simulink model "ros2webots_localization_model_cg"  (R2023a)
settings: Solver=FixedStepDiscrete  StartTime=0.0  StopTime=inf  FixedStep=0.05  RelTol=1e-3  EnableMultiTasking=on
model workspace (MAT data in the model file):
  Logfile_Data_Object = robotics.ros.BagSelection
  Logfile_Data_Object.FilePath = '\\wsl.localhost\ubuntu\home\mjavadzallaghi\ros2_ws\ros2webots\baglog\rosbot_data_20240125_225927.bag'
  Logfile_Data_Object.StartTime = 1706210981.23
  Logfile_Data_Object.EndTime = 1706211126.25
  Logfile_Data_Object.NumMessages = 508
  Logfile_Data_Object.AvailableTopics = table
  Logfile_Data_Object.AvailableTopics.data{1} = [73; 435]
  Logfile_Data_Object.AvailableTopics.data{2} = categorical
  Logfile_Data_Object.AvailableTopics.data{2}.categoryNames = {'geometry_msgs/Twist'; 'sensor_msgs/Imu'}
  Logfile_Data_Object.AvailableTopics.data{2}.codes = [1; 2]
  Logfile_Data_Object.AvailableTopics.data{3}{1} = 'geometry_msgs/Vector3 Linear
    |   double X
    |   double Y
    |   double Z
    | geometry_msgs/Vector3 Angular
    |   double X
    |   double Y
    |   double Z
    | '
  Logfile_Data_Object.AvailableTopics.data{3}{2} = 'std_msgs/Header Header
    |   uint32 Seq
    |   Time Stamp
    |   char FrameId
    | geometry_msgs/Quaternion Orientation
    |   double X
    |   double Y
    |   double Z
    |   double W
    | double[9] OrientationCovariance
    | geometry_msgs/Vector3 AngularVelocity
    |   double X
    |   double Y
    |   double Z
    | double[9] AngularVelocityCovariance
    | geometry_msgs/Vector3 LinearAcceleration
    |   double X
    |   double Y
    |   double Z
    | double[9] LinearAccelerationCovariance
    | '
  Logfile_Data_Object.AvailableTopics.ndims = 2
  Logfile_Data_Object.AvailableTopics.nrows = 2
  Logfile_Data_Object.AvailableTopics.rownames = {'/webots/rosbot/command_vel'; '/webots/rosbot/imu'}
  Logfile_Data_Object.AvailableTopics.nvars = 3
  Logfile_Data_Object.AvailableTopics.varnames = {'NumMessages', 'MessageType', 'MessageDefinition'}
  Logfile_Data_Object.AvailableTopics.props.useVariableNamesOriginal = 0
  Logfile_Data_Object.AvailableTopics.props.useDimensionNamesOriginal = 0
  Logfile_Data_Object.AvailableTopics.props.CustomProps = struct()
  Logfile_Data_Object.AvailableTopics.props.VariableCustomProps = struct()
  Logfile_Data_Object.AvailableTopics.props.versionSavedFrom = 4
  Logfile_Data_Object.AvailableTopics.props.minCompatibleVersion = 1
  Logfile_Data_Object.AvailableTopics.props.incompatibilityMsg = ''
  Logfile_Data_Object.AvailableTopics.props.VersionSavedFrom = 4
  Logfile_Data_Object.AvailableTopics.props.Description = ''
  Logfile_Data_Object.AvailableTopics.props.VariableNamesOriginal = {}
  Logfile_Data_Object.AvailableTopics.props.DimensionNames = {'Row', 'Variables'}
  Logfile_Data_Object.AvailableTopics.props.DimensionNamesOriginal = {}
  Logfile_Data_Object.AvailableTopics.props.UserData = []
  Logfile_Data_Object.AvailableTopics.props.VariableDescriptions = {}
  Logfile_Data_Object.AvailableTopics.props.VariableUnits = {}
  Logfile_Data_Object.AvailableTopics.props.VariableContinuity = {}
  Logfile_Data_Object.MessageList = table
  Logfile_Data_Object.MessageList.data{1} = [1706210981.23 1706210981.23 1706210981.23 1706210983.05 1706210983.38 1706210983.7 1706210984.04 1706210984.38 1706210984.72 1706210985.07 1706210985.41 1706210985.73 ... (508 elements, 508x1)]
  Logfile_Data_Object.MessageList.data{2} = categorical
  Logfile_Data_Object.MessageList.data{2}.categoryNames = {'/webots/rosbot/command_vel'; '/webots/rosbot/imu'}
  Logfile_Data_Object.MessageList.data{2}.codes = [1; 1; 1; 2; 2; 2; 2; 2; 2; 2; 2; 1; 1; 1; 2; 2; 2; 2; 2; 2; 2; 2; 2; 2; 2; 2; 2; 2; 2; 2; 2; 2; 2; 2; 2; 2; 2; 2; 1; 1; 1; 2; 2; 2; 2; 2; 2; 2; 2; 2; 2; 2; 2; 2; 2; 2; 2; 2; 2; 2; 2; 2; 2; 2; 2; 2; 2; 1; 1; 1; 2; 2; 2; 2; 2; 2; 2; 2; 2; 2; 2; 2; 2; 2; 2; 2; 2; 2; 2; 2; 2; 1; 1; 1; 2; 2; 2; 2; 2; 2; 2; 2; 2; 2; 2; 2; 2; 2; 2; 2; 2; 2; 2; 2; 2; 2; 2; 2; 1; 1; 2; 1; 2; 2; 2; 2; 2; 2; 2; 2; 2; 2; 2; 2; 2; 2; 2; 2; 2; 2; 2; 2; 2; 2; 2; 2; 2; 2; 2; 2; 2; 2; 2; 2; 2; 2; 2; 2; 2; 2; 2; 2; 2; 2; 2; 2; 1; 1; 1; 2; 2; 2; 2; 2; 2; 2; 2; 2; 2; 2; 2; 2; 2; 2; 2; 2; 2; 2; 2; 2; 2; 2; 2; 1; 1; 1; 2; 2; 2; 2; 2; 2; 2; 2; 2; 2; 2; 2; 2; 2; 2; 2; 2; 2; 2; 2; 2; 2; 2; 2; 2; 2; 2; 1; 1; 1; 2; 2; 2; 2; 2; 2; 2; 2; 2; 2; 2; 2; 2; 2; 2; 2; 2; 2; 2; 2; 2; 2; 2; 2; 2; 2; 1; 1; 1; 2; 2; 2; 2; 2; 2; 2; 2; 2; 2; 2; 2; 2; 2; 2; 2; 2; 2; 2; 2; 1; 1; 1; 2; 2; 2; 2; 2; 2; 2; 2; 2; 2; 2; 2; 2; 2; 2; 2; 2; 2; 2; 2; 2; 2; 2; 2; 2; 1; 1; 1; 2; 2; 2; 2; 2; 2; 2; 1; 1; 2; 1; 2; 2; 2; 2; 2; 2; 1; 1; 1; 2; 2; 2; 2; 2; 2; 2; 2; 2; 2; 2; 2; 1; 1; 1; 2; 2; 2; 2; 2; 2; 2; 2; 2; 2; 2; 2; 2; 2; 2; 2; 2; 2; 2; 1; 1; 1; 2; 2; 2; 2; 2; 2; 2; 2; 2; 1; 1; 1; 2; 2; 2; 2; 2; 2; 2; 2; 2; 2; 2; 2; 1; 1; 1; 2; 2; 2; 2; 2; 2; 1; 1; 1; 2; 2; 2; 2; 2; 2; 2; 2; 2; 2; 2; 2; 1; 1; 1; 2; 2; 2; 2; 2; 2; 2; 2; 2; 2; 1; 1; 1; 2; 2; 2; 2; 2; 2; 2; 2; 2; 2; 1; 1; 1; 2; 2; 2; 2; 2; 2; 2; 1; 1; 1; 2; 2; 2; 2; 2; 2; 2; 2; 2; 2; 2; 2; 2; 2; 2; 2; 1; 1; 1; 2; 2; 2; 2; 2; 2; 2; 2; 2; 2; 2; 2; 2; 2; 2; 2; 1; 2; 2; 2; 2; 2; 2; 2; 2; 2; 2; 2; 2; 2; 2; 2; 2; 2; 2; 2; 2; 2; 2]
  Logfile_Data_Object.MessageList.data{3} = categorical
  Logfile_Data_Object.MessageList.data{3}.categoryNames = {'geometry_msgs/Twist'; 'sensor_msgs/Imu'}
  Logfile_Data_Object.MessageList.data{3}.codes = [1; 1; 1; 2; 2; 2; 2; 2; 2; 2; 2; 1; 1; 1; 2; 2; 2; 2; 2; 2; 2; 2; 2; 2; 2; 2; 2; 2; 2; 2; 2; 2; 2; 2; 2; 2; 2; 2; 1; 1; 1; 2; 2; 2; 2; 2; 2; 2; 2; 2; 2; 2; 2; 2; 2; 2; 2; 2; 2; 2; 2; 2; 2; 2; 2; 2; 2; 1; 1; 1; 2; 2; 2; 2; 2; 2; 2; 2; 2; 2; 2; 2; 2; 2; 2; 2; 2; 2; 2; 2; 2; 1; 1; 1; 2; 2; 2; 2; 2; 2; 2; 2; 2; 2; 2; 2; 2; 2; 2; 2; 2; 2; 2; 2; 2; 2; 2; 2; 1; 1; 2; 1; 2; 2; 2; 2; 2; 2; 2; 2; 2; 2; 2; 2; 2; 2; 2; 2; 2; 2; 2; 2; 2; 2; 2; 2; 2; 2; 2; 2; 2; 2; 2; 2; 2; 2; 2; 2; 2; 2; 2; 2; 2; 2; 2; 2; 1; 1; 1; 2; 2; 2; 2; 2; 2; 2; 2; 2; 2; 2; 2; 2; 2; 2; 2; 2; 2; 2; 2; 2; 2; 2; 2; 1; 1; 1; 2; 2; 2; 2; 2; 2; 2; 2; 2; 2; 2; 2; 2; 2; 2; 2; 2; 2; 2; 2; 2; 2; 2; 2; 2; 2; 2; 1; 1; 1; 2; 2; 2; 2; 2; 2; 2; 2; 2; 2; 2; 2; 2; 2; 2; 2; 2; 2; 2; 2; 2; 2; 2; 2; 2; 2; 1; 1; 1; 2; 2; 2; 2; 2; 2; 2; 2; 2; 2; 2; 2; 2; 2; 2; 2; 2; 2; 2; 2; 1; 1; 1; 2; 2; 2; 2; 2; 2; 2; 2; 2; 2; 2; 2; 2; 2; 2; 2; 2; 2; 2; 2; 2; 2; 2; 2; 2; 1; 1; 1; 2; 2; 2; 2; 2; 2; 2; 1; 1; 2; 1; 2; 2; 2; 2; 2; 2; 1; 1; 1; 2; 2; 2; 2; 2; 2; 2; 2; 2; 2; 2; 2; 1; 1; 1; 2; 2; 2; 2; 2; 2; 2; 2; 2; 2; 2; 2; 2; 2; 2; 2; 2; 2; 2; 1; 1; 1; 2; 2; 2; 2; 2; 2; 2; 2; 2; 1; 1; 1; 2; 2; 2; 2; 2; 2; 2; 2; 2; 2; 2; 2; 1; 1; 1; 2; 2; 2; 2; 2; 2; 1; 1; 1; 2; 2; 2; 2; 2; 2; 2; 2; 2; 2; 2; 2; 1; 1; 1; 2; 2; 2; 2; 2; 2; 2; 2; 2; 2; 1; 1; 1; 2; 2; 2; 2; 2; 2; 2; 2; 2; 2; 1; 1; 1; 2; 2; 2; 2; 2; 2; 2; 1; 1; 1; 2; 2; 2; 2; 2; 2; 2; 2; 2; 2; 2; 2; 2; 2; 2; 2; 1; 1; 1; 2; 2; 2; 2; 2; 2; 2; 2; 2; 2; 2; 2; 2; 2; 2; 2; 1; 2; 2; 2; 2; 2; 2; 2; 2; 2; 2; 2; 2; 2; 2; 2; 2; 2; 2; 2; 2; 2; 2]
  Logfile_Data_Object.MessageList.data{4} = [5438 5532 5626 5720 6078 6436 6794 7152 7510 7868 8226 8584 ... (508 elements, 508x1)]
  Logfile_Data_Object.MessageList.ndims = 2
  Logfile_Data_Object.MessageList.nrows = 508
  Logfile_Data_Object.MessageList.nvars = 4
  Logfile_Data_Object.MessageList.varnames = {'Time', 'Topic', 'MessageType', 'FileOffset'}
  Logfile_Data_Object.MessageList.props.useVariableNamesOriginal = 0
  Logfile_Data_Object.MessageList.props.useDimensionNamesOriginal = 0
  Logfile_Data_Object.MessageList.props.CustomProps = struct()
  Logfile_Data_Object.MessageList.props.VariableCustomProps = struct()
  Logfile_Data_Object.MessageList.props.versionSavedFrom = 4
  Logfile_Data_Object.MessageList.props.minCompatibleVersion = 1
  Logfile_Data_Object.MessageList.props.incompatibilityMsg = ''
  Logfile_Data_Object.MessageList.props.VersionSavedFrom = 4
  Logfile_Data_Object.MessageList.props.Description = ''
  Logfile_Data_Object.MessageList.props.VariableNamesOriginal = {}
  Logfile_Data_Object.MessageList.props.DimensionNames = {'Row', 'Variables'}
  Logfile_Data_Object.MessageList.props.DimensionNamesOriginal = {}
  Logfile_Data_Object.MessageList.props.UserData = []
  Logfile_Data_Object.MessageList.props.VariableDescriptions = {}
  Logfile_Data_Object.MessageList.props.VariableUnits = {}
  Logfile_Data_Object.MessageList.props.VariableContinuity = {}
  Logfile_Data_Object.RawMessageBuffer = containers.Map
  Logfile_Data_Object.RawMessageBuffer.serialization.keys = {}
  Logfile_Data_Object.RawMessageBuffer.serialization.values = {}
  Logfile_Data_Object.RawMessageBuffer.serialization.uniformity = 0
  Logfile_Data_Object.RawMessageBuffer.serialization.keyType = 'char'
  Logfile_Data_Object.RawMessageBuffer.serialization.valueType = 'any'
  Logfile_Data_Object.ImgMessageBuffer = containers.Map
  Logfile_Data_Object.ImgMessageBuffer.serialization.keys = {}
  Logfile_Data_Object.ImgMessageBuffer.serialization.values = {}
  Logfile_Data_Object.ImgMessageBuffer.serialization.uniformity = 0
  Logfile_Data_Object.ImgMessageBuffer.serialization.keyType = 'char'
  Logfile_Data_Object.ImgMessageBuffer.serialization.valueType = 'any'
  Logfile_Data_Object.PointCloudBuffer = containers.Map
  Logfile_Data_Object.PointCloudBuffer.serialization.keys = {}
  Logfile_Data_Object.PointCloudBuffer.serialization.values = {}
  Logfile_Data_Object.PointCloudBuffer.serialization.uniformity = 0
  Logfile_Data_Object.PointCloudBuffer.serialization.keyType = 'char'
  Logfile_Data_Object.PointCloudBuffer.serialization.valueType = 'any'
  Logfile_Data_Object.LaserScanBuffer = containers.Map
  Logfile_Data_Object.LaserScanBuffer.serialization.keys = {}
  Logfile_Data_Object.LaserScanBuffer.serialization.values = {}
  Logfile_Data_Object.LaserScanBuffer.serialization.uniformity = 0
  Logfile_Data_Object.LaserScanBuffer.serialization.keyType = 'char'
  Logfile_Data_Object.LaserScanBuffer.serialization.valueType = 'any'
  Logfile_Data_Object.TopicTypeMap = containers.Map
  Logfile_Data_Object.TopicTypeMap.serialization.keys = {'/webots/rosbot/command_vel', '/webots/rosbot/imu'}
  Logfile_Data_Object.TopicTypeMap.serialization.values = {'geometry_msgs/Twist', 'sensor_msgs/Imu'}
  Logfile_Data_Object.TopicTypeMap.serialization.uniformity = 1
  Logfile_Data_Object.TopicTypeMap.serialization.keyType = 'char'
  Logfile_Data_Object.TopicTypeMap.serialization.valueType = 'char'
  Logfile_Data_Object.TopicDefinitionMap = containers.Map
  Logfile_Data_Object.TopicDefinitionMap.serialization.keys = {'/webots/rosbot/command_vel', '/webots/rosbot/imu'}
  Logfile_Data_Object.TopicDefinitionMap.serialization.values{1} = 'geometry_msgs/Vector3 Linear
    |   double X
    |   double Y
    |   double Z
    | geometry_msgs/Vector3 Angular
    |   double X
    |   double Y
    |   double Z
    | '
  Logfile_Data_Object.TopicDefinitionMap.serialization.values{2} = 'std_msgs/Header Header
    |   uint32 Seq
    |   Time Stamp
    |   char FrameId
    | geometry_msgs/Quaternion Orientation
    |   double X
    |   double Y
    |   double Z
    |   double W
    | double[9] OrientationCovariance
    | geometry_msgs/Vector3 AngularVelocity
    |   double X
    |   double Y
    |   double Z
    | double[9] AngularVelocityCovariance
    | geometry_msgs/Vector3 LinearAcceleration
    |   double X
    |   double Y
    |   double Z
    | double[9] LinearAccelerationCovariance
    | '
  Logfile_Data_Object.TopicDefinitionMap.serialization.uniformity = 1
  Logfile_Data_Object.TopicDefinitionMap.serialization.keyType = 'char'
  Logfile_Data_Object.TopicDefinitionMap.serialization.valueType = 'char'
  Logfile_Data_Object.messageTypeMap = containers.Map
  Logfile_Data_Object.messageTypeMap.serialization.keys = {}
  Logfile_Data_Object.messageTypeMap.serialization.values = {}
  Logfile_Data_Object.messageTypeMap.serialization.uniformity = 0
  Logfile_Data_Object.messageTypeMap.serialization.keyType = 'char'
  Logfile_Data_Object.messageTypeMap.serialization.valueType = 'any'
  Logfile_Data_Object.Parser = robotics.ros.internal.tf.TransformationTreeParser
  Logfile_Data_Object.Parser.UseObjectMsg = 1
  Logfile_Path = '\\wsl.localhost\ubuntu\home\mjavadzallaghi\ros2_ws\ros2webots\baglog\rosbot_data_20240125_225927.bag'
  Logfile_Playback_Duration = nan
  Logfile_Playback_Offset = nan
values from neighbouring files (symbols this model uses):
  wheel_based_localization_x_initial_coord = 0.0    [ros2webots_localization_model.sldd]
  wheel_based_localization_y_initial_coord = 0.0    [ros2webots_localization_model.sldd]
libraries: sharedtransform x1
settings Model: DataDictionary=ros2webots_localization_model.sldd  Creator=MJava  LastModifiedBy=MJava
settings SolverCC: AllowMultiTaskInputOutput=on  AutoInsertRateTranBlk=on
settings OptimizationCC: DefaultParameterBehavior=Inlined  EnhancedBackFolding=on  PassReuseOutputArgsAs=Individual arguments  ZeroExternalMemoryAtStartup=off  ZeroInternalMemoryAtStartup=off  MaxStackSize=64  OptimizeBlockOrder=speed  DifferentSizesBufferReuse=on  OptimizationCustomize=off  EfficientTunableParamExpr=on
settings DebuggingCC: ParameterTunabilityLossMsg=error
settings SFSimCC: MATLABDynamicMemAlloc=off  SimTargetLang=C++
settings RTWCC: Description=Embedded Coder  SystemTargetFile=ert.tlc  TemplateMakefile=ert_default_tmf  GenerateReport=on  Toolchain=Microsoft Visual C++ 2019 v16.0 | nmake (64-bit Windows)  BuildConfiguration=Faster Runs  LaunchReport=on  TargetLang=C++  GenerateWebview=on  GenerateCodeMetricsReport=on  CheckMdlBeforeBuild=Warning
settings CodeAppCC: ForceParamTrailComments=on  IgnoreCustomStorageClasses=off  OperatorAnnotations=on  SimulinkDataObjDesc=on  SFDataObjDesc=on  InsertBlockDesc=on
settings ERTTargetCC: TargetLangStandard=C++11 (ISO)  CodeInterfacePackaging=C++ class  RootIOFormat=Structure reference  ERTCustomFileTemplate=example_file_process.tlc

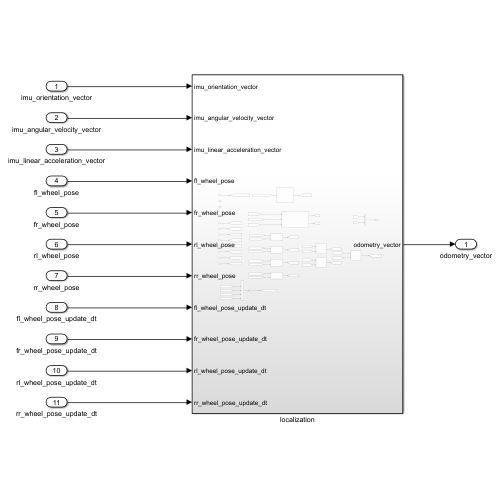
[thumbnail: Simulink's stored preview of the top-level diagram]
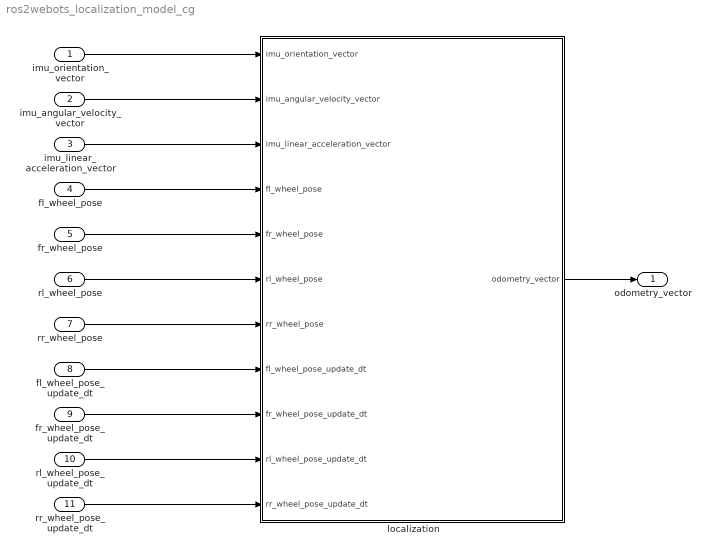
== system ros2webots_localization_model_cg ==
  imu_orientation_vector : Inport  OutDataTypeStr=double  PortDimensions=4
  imu_angular_velocity_vector : Inport  Port=2  OutDataTypeStr=double  PortDimensions=3
  imu_linear_acceleration_vector : Inport  Port=3  OutDataTypeStr=double  PortDimensions=3
  fl_wheel_pose : Inport  Port=4  OutDataTypeStr=double  PortDimensions=1
  fr_wheel_pose : Inport  Port=5  OutDataTypeStr=double  PortDimensions=1
  rl_wheel_pose : Inport  Port=6  OutDataTypeStr=double  PortDimensions=1
  rr_wheel_pose : Inport  Port=7  OutDataTypeStr=double  PortDimensions=1
  fl_wheel_pose_update_dt : Inport  Port=8  OutDataTypeStr=double  PortDimensions=1
  fr_wheel_pose_update_dt : Inport  Port=9  OutDataTypeStr=double  PortDimensions=1
  rl_wheel_pose_update_dt : Inport  Port=10  OutDataTypeStr=double  PortDimensions=1
  rr_wheel_pose_update_dt : Inport  Port=11  OutDataTypeStr=double  PortDimensions=1
  localization : Subsystem
  odometry_vector : Outport  OutDataTypeStr=double  PortDimensions=2
  wires:
  imu_orientation_vector/1 -> localization/1(imu_orientation_vector)
  imu_linear_acceleration_vector/1 -> localization/3(imu_linear_acceleration_vector)
  imu_angular_velocity_vector/1 -> localization/2(imu_angular_velocity_vector)
  rl_wheel_pose/1 -> localization/6(rl_wheel_pose)
  rr_wheel_pose/1 -> localization/7(rr_wheel_pose)
  fl_wheel_pose/1 -> localization/4(fl_wheel_pose)
  fr_wheel_pose/1 -> localization/5(fr_wheel_pose)
  rl_wheel_pose_update_dt/1 -> localization/10(rl_wheel_pose_update_dt)
  fr_wheel_pose_update_dt/1 -> localization/9(fr_wheel_pose_update_dt)
  fl_wheel_pose_update_dt/1 -> localization/8(fl_wheel_pose_update_dt)
  rr_wheel_pose_update_dt/1 -> localization/11(rr_wheel_pose_update_dt)
  localization/1(odometry_vector) -> odometry_vector/1

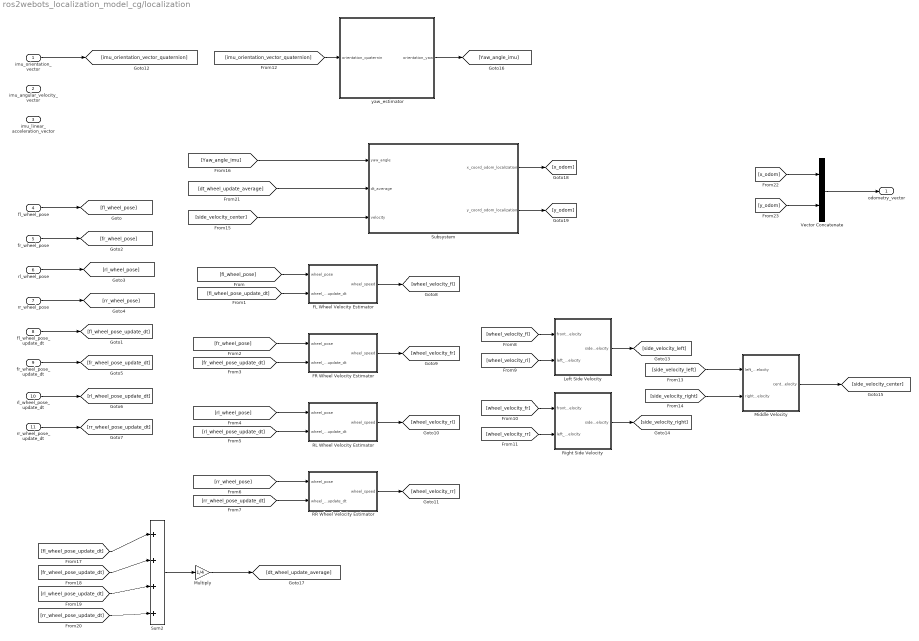
== system ros2webots_localization_model_cg/localization ==
  imu_orientation_vector : Inport  OutDataTypeStr=double  PortDimensions=4
  imu_angular_velocity_vector : Inport  Port=2  OutDataTypeStr=double  PortDimensions=3
  imu_linear_acceleration_vector : Inport  Port=3  OutDataTypeStr=double  PortDimensions=3
  fl_wheel_pose : Inport  Port=4
  fr_wheel_pose : Inport  Port=5
  rl_wheel_pose : Inport  Port=6
  rr_wheel_pose : Inport  Port=7
  fl_wheel_pose_update_dt : Inport  Port=8
  fr_wheel_pose_update_dt : Inport  Port=9
  rl_wheel_pose_update_dt : Inport  Port=10
  rr_wheel_pose_update_dt : Inport  Port=11
  FL Wheel Velocity Estimator : Subsystem
  FR Wheel Velocity Estimator : Subsystem
  Left Side Velocity : Subsystem
  Middle Velocity : Subsystem
  Multiply : Gain  Gain=1/4
  RL Wheel Velocity Estimator : Subsystem
  RR Wheel Velocity Estimator : Subsystem
  Right Side Velocity : Subsystem
  Subsystem : Subsystem
  Sum2 : Sum  Inputs=|++++
  Vector Concatenate : Concatenate
  yaw_estimator : Subsystem
  odometry_vector : Outport  PortDimensions=2
  wires:
  fl_wheel_pose_update_dt/1 -> [fl_wheel_pose_update_dt]
  [fl_wheel_pose] -> FL Wheel Velocity Estimator/1(wheel_pose)
  [fl_wheel_pose_update_dt] -> FL Wheel Velocity Estimator/2(wheel_pose_update_dt)
  fl_wheel_pose/1 -> [fl_wheel_pose]
  fr_wheel_pose/1 -> [fr_wheel_pose]
  rl_wheel_pose/1 -> [rl_wheel_pose]
  rr_wheel_pose/1 -> [rr_wheel_pose]
  fr_wheel_pose_update_dt/1 -> [fr_wheel_pose_update_dt]
  rl_wheel_pose_update_dt/1 -> [rl_wheel_pose_update_dt]
  rr_wheel_pose_update_dt/1 -> [rr_wheel_pose_update_dt]
  [fr_wheel_pose] -> FR Wheel Velocity Estimator/1(wheel_pose)
  [fr_wheel_pose_update_dt] -> FR Wheel Velocity Estimator/2(wheel_pose_update_dt)
  [rl_wheel_pose] -> RL Wheel Velocity Estimator/1(wheel_pose)
  [rl_wheel_pose_update_dt] -> RL Wheel Velocity Estimator/2(wheel_pose_update_dt)
  [rr_wheel_pose] -> RR Wheel Velocity Estimator/1(wheel_pose)
  [rr_wheel_pose_update_dt] -> RR Wheel Velocity Estimator/2(wheel_pose_update_dt)
  FL Wheel Velocity Estimator/1(wheel_speed) -> [wheel_velocity_fl]
  FR Wheel Velocity Estimator/1(wheel_speed) -> [wheel_velocity_fr]
  RL Wheel Velocity Estimator/1(wheel_speed) -> [wheel_velocity_rl]
  RR Wheel Velocity Estimator/1(wheel_speed) -> [wheel_velocity_rr]
  [wheel_velocity_fl] -> Left Side Velocity/1(front_wheel_velocity)
  [wheel_velocity_rl] -> Left Side Velocity/2(left_wheel_velocity)
  [wheel_velocity_fr] -> Right Side Velocity/1(front_wheel_velocity)
  [wheel_velocity_rr] -> Right Side Velocity/2(left_wheel_velocity)
  imu_orientation_vector/1 -> [imu_orientation_vector_quaternion]
  [imu_orientation_vector_quaternion] -> yaw_estimator/1(orientation_quaternin)
  Left Side Velocity/1(side_velocity) -> [side_velocity_left]
  Right Side Velocity/1(side_velocity) -> [side_velocity_right]
  [side_velocity_left] -> Middle Velocity/1(left_side_velocity)
  [side_velocity_right] -> Middle Velocity/2(right_side_velocity)
  Middle Velocity/1(center_velocity) -> [side_velocity_center]
  yaw_estimator/1(orientation_yaw) -> [Yaw_angle_imu]
  [fl_wheel_pose_update_dt] -> Sum2/1
  [fr_wheel_pose_update_dt] -> Sum2/2
  [rl_wheel_pose_update_dt] -> Sum2/3
  [rr_wheel_pose_update_dt] -> Sum2/4
  Sum2/1 -> Multiply/1
  Multiply/1 -> [dt_wheel_update_average]
  [dt_wheel_update_average] -> Subsystem/2(dt_average)
  [side_velocity_center] -> Subsystem/3(velocity)
  Subsystem/1(x_coord_odom_localization) -> [x_odom]
  Subsystem/2(y_coord_odom_localization) -> [y_odom]
  [x_odom] -> Vector Concatenate/1
  [y_odom] -> Vector Concatenate/2
  Vector Concatenate/1 -> odometry_vector/1
  [Yaw_angle_imu] -> Subsystem/1(yaw_angle)

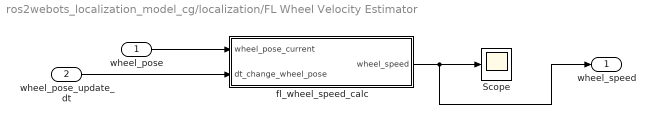
== system ros2webots_localization_model_cg/localization/FL Wheel Velocity Estimator ==
  wheel_pose : Inport
  wheel_pose_update_dt : Inport  Port=2
  Scope : Scope
  fl_wheel_speed_calc : Subsystem
  wheel_speed : Outport
  wires:
  wheel_pose/1 -> fl_wheel_speed_calc/1(wheel_pose_current)
  fl_wheel_speed_calc/1(wheel_speed) -> wheel_speed/1, Scope/1
  wheel_pose_update_dt/1 -> fl_wheel_speed_calc/2(dt_change_wheel_pose)

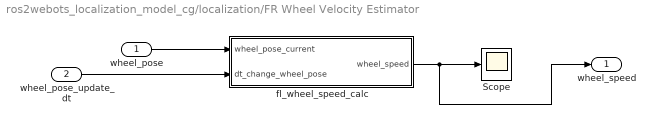
== system ros2webots_localization_model_cg/localization/FR Wheel Velocity Estimator ==
  wheel_pose : Inport
  wheel_pose_update_dt : Inport  Port=2
  Scope : Scope
  fl_wheel_speed_calc : Subsystem
  wheel_speed : Outport
  wires:
  wheel_pose/1 -> fl_wheel_speed_calc/1(wheel_pose_current)
  fl_wheel_speed_calc/1(wheel_speed) -> wheel_speed/1, Scope/1
  wheel_pose_update_dt/1 -> fl_wheel_speed_calc/2(dt_change_wheel_pose)

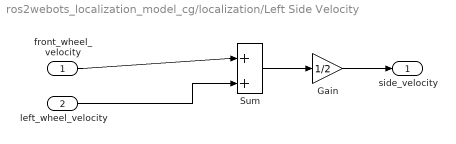
== system ros2webots_localization_model_cg/localization/Left Side Velocity ==
  front_wheel_velocity : Inport
  left_wheel_velocity : Inport  Port=2
  Gain : Gain  Gain=1/2
  Sum : Sum  Inputs=|++
  side_velocity : Outport
  wires:
  left_wheel_velocity/1 -> Sum/2
  front_wheel_velocity/1 -> Sum/1
  Sum/1 -> Gain/1
  Gain/1 -> side_velocity/1

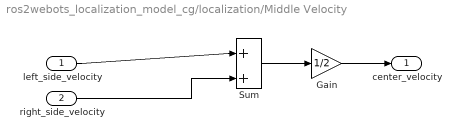
== system ros2webots_localization_model_cg/localization/Middle Velocity ==
  left_side_velocity : Inport
  right_side_velocity : Inport  Port=2
  Gain : Gain  Gain=1/2
  Sum : Sum  Inputs=|++
  center_velocity : Outport
  wires:
  right_side_velocity/1 -> Sum/2
  left_side_velocity/1 -> Sum/1
  Sum/1 -> Gain/1
  Gain/1 -> center_velocity/1

== system ros2webots_localization_model_cg/localization/RL Wheel Velocity Estimator ==
  wheel_pose : Inport
  wheel_pose_update_dt : Inport  Port=2
  Scope : Scope
  fl_wheel_speed_calc : Subsystem
  wheel_speed : Outport
  wires:
  wheel_pose/1 -> fl_wheel_speed_calc/1(wheel_pose_current)
  fl_wheel_speed_calc/1(wheel_speed) -> wheel_speed/1, Scope/1
  wheel_pose_update_dt/1 -> fl_wheel_speed_calc/2(dt_change_wheel_pose)

== system ros2webots_localization_model_cg/localization/RR Wheel Velocity Estimator ==
  wheel_pose : Inport
  wheel_pose_update_dt : Inport  Port=2
  Scope : Scope
  fl_wheel_speed_calc : Subsystem
  wheel_speed : Outport
  wires:
  wheel_pose/1 -> fl_wheel_speed_calc/1(wheel_pose_current)
  fl_wheel_speed_calc/1(wheel_speed) -> wheel_speed/1, Scope/1
  wheel_pose_update_dt/1 -> fl_wheel_speed_calc/2(dt_change_wheel_pose)

== system ros2webots_localization_model_cg/localization/Right Side Velocity ==
  front_wheel_velocity : Inport
  left_wheel_velocity : Inport  Port=2
  Gain : Gain  Gain=1/2
  Sum : Sum  Inputs=|++
  side_velocity : Outport
  wires:
  left_wheel_velocity/1 -> Sum/2
  front_wheel_velocity/1 -> Sum/1
  Sum/1 -> Gain/1
  Gain/1 -> side_velocity/1

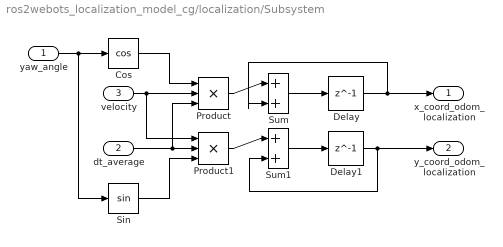
== system ros2webots_localization_model_cg/localization/Subsystem ==
  yaw_angle : Inport
  dt_average : Inport  Port=2
  velocity : Inport  Port=3
  Cos : Trigonometry  Operator=cos
  Delay : Delay  DelayLength=1  InitialCondition=wheel_based_localization_x_initial_coord
  Delay1 : Delay  DelayLength=1  InitialCondition=wheel_based_localization_y_initial_coord
  Product : Product  Inputs=3  OutDataTypeStr=double
  Product1 : Product  Inputs=3
  Sin : Trigonometry
  Sum : Sum  Inputs=|++
  Sum1 : Sum  Inputs=|++
  x_coord_odom_localization : Outport
  y_coord_odom_localization : Outport  Port=2
  wires:
  yaw_angle/1 -> Sin/1, Cos/1
  dt_average/1 -> Product1/2, Product/3
  Delay1/1 -> y_coord_odom_localization/1, Sum1/2
  Cos/1 -> Product/1
  Product1/1 -> Sum1/1
  Product/1 -> Sum/1
  velocity/1 -> Product/2, Product1/1
  Sin/1 -> Product1/3
  Sum/1 -> Delay/1
  Sum1/1 -> Delay1/1
  Delay/1 -> Sum/2, x_coord_odom_localization/1

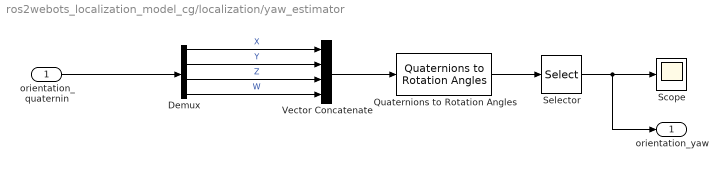
== system ros2webots_localization_model_cg/localization/yaw_estimator ==
  orientation_quaternin : Inport
  Demux : Demux
  Quaternions to Rotation Angles : sharedtransform/Quaternions to Rotation Angles  rotationOrder=ZYX  aMode=aMode
  Scope : Scope
  Selector : Selector  InputPortWidth=3  IndexOptions=Index vector (dialog)  Indices=3  OutputSizes=1
  Vector Concatenate : Concatenate  NumInputs=4
  orientation_yaw : Outport
  wires:
  Quaternions to Rotation Angles/1 -> Selector/1
  orientation_quaternin/1 -> Demux/1
  Selector/1 -> orientation_yaw/1, Scope/1
  Vector Concatenate/1 -> Quaternions to Rotation Angles/1
  Demux/1 -> Vector Concatenate/1  "X"
  Demux/2 -> Vector Concatenate/2  "Y"
  Demux/3 -> Vector Concatenate/3  "Z"
  Demux/4 -> Vector Concatenate/4  "W"

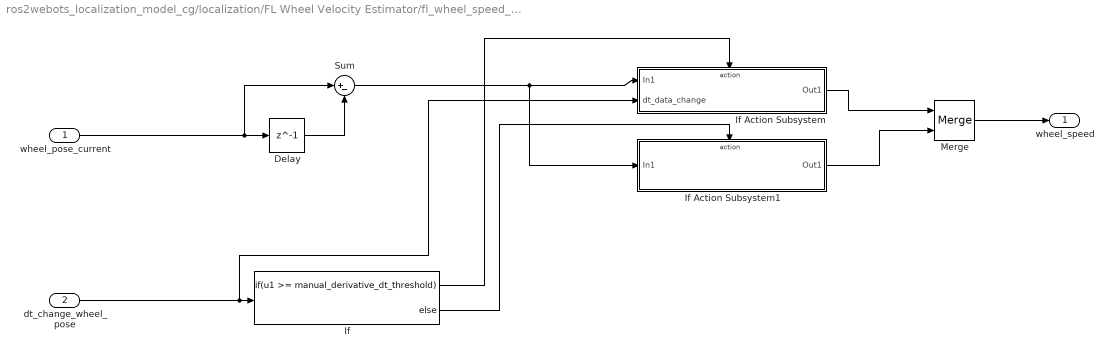
== system ros2webots_localization_model_cg/localization/FL Wheel Velocity Estimator/fl_wheel_speed_calc ==
  wheel_pose_current : Inport
  dt_change_wheel_pose : Inport  Port=2
  Delay : Delay  DelayLength=1
  If : If  IfExpression=u1 >= manual_derivative_dt_threshold
  If Action Subsystem : Subsystem  TreatAsAtomicUnit=on
  If Action Subsystem1 : Subsystem  TreatAsAtomicUnit=on
  Merge : Merge
  Sum : Sum  Inputs=|+-
  wheel_speed : Outport
  wires:
  Sum/1 -> If Action Subsystem/1(In1), If Action Subsystem1/1(In1)
  Delay/1 -> Sum/2
  dt_change_wheel_pose/1 -> If/1, If Action Subsystem/2(dt_data_change)
  If Action Subsystem/1(Out1) -> Merge/1
  If Action Subsystem1/1(Out1) -> Merge/2
  wheel_pose_current/1 -> Sum/1, Delay/1
  If/2 -> If Action Subsystem1/Action
  If/1 -> If Action Subsystem/Action
  Merge/1 -> wheel_speed/1

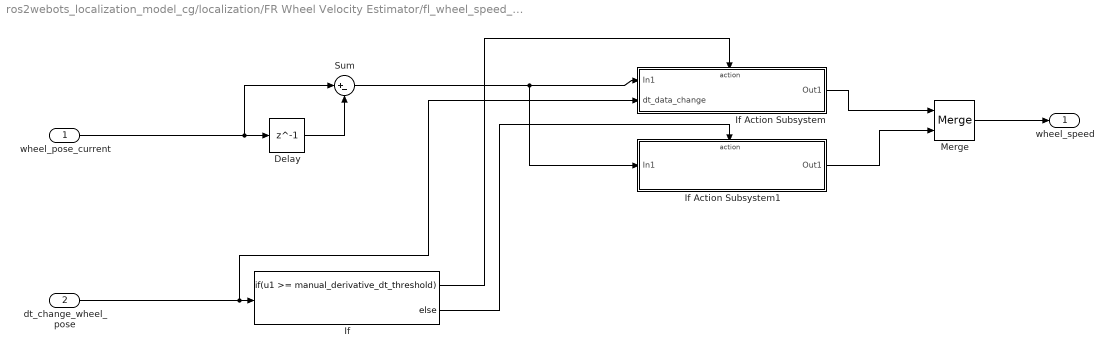
== system ros2webots_localization_model_cg/localization/FR Wheel Velocity Estimator/fl_wheel_speed_calc ==
  wheel_pose_current : Inport
  dt_change_wheel_pose : Inport  Port=2
  Delay : Delay  DelayLength=1
  If : If  IfExpression=u1 >= manual_derivative_dt_threshold
  If Action Subsystem : Subsystem  TreatAsAtomicUnit=on
  If Action Subsystem1 : Subsystem  TreatAsAtomicUnit=on
  Merge : Merge
  Sum : Sum  Inputs=|+-
  wheel_speed : Outport
  wires:
  Sum/1 -> If Action Subsystem/1(In1), If Action Subsystem1/1(In1)
  Delay/1 -> Sum/2
  dt_change_wheel_pose/1 -> If/1, If Action Subsystem/2(dt_data_change)
  If Action Subsystem/1(Out1) -> Merge/1
  If Action Subsystem1/1(Out1) -> Merge/2
  wheel_pose_current/1 -> Sum/1, Delay/1
  If/2 -> If Action Subsystem1/Action
  If/1 -> If Action Subsystem/Action
  Merge/1 -> wheel_speed/1

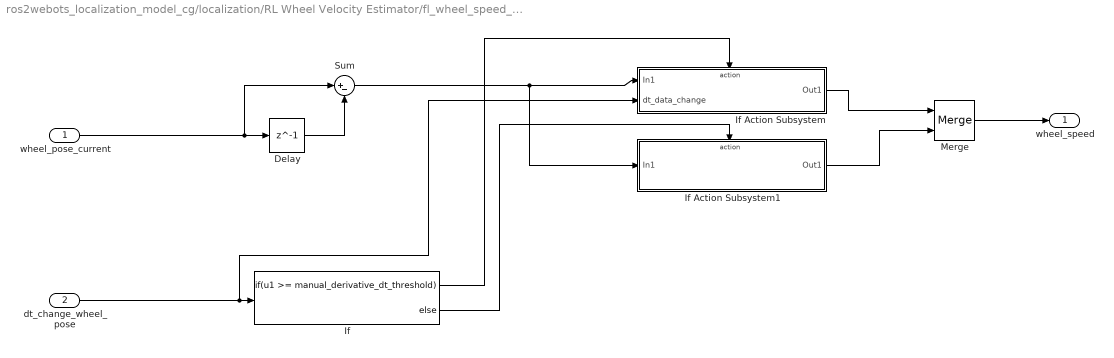
== system ros2webots_localization_model_cg/localization/RL Wheel Velocity Estimator/fl_wheel_speed_calc ==
  wheel_pose_current : Inport
  dt_change_wheel_pose : Inport  Port=2
  Delay : Delay  DelayLength=1
  If : If  IfExpression=u1 >= manual_derivative_dt_threshold
  If Action Subsystem : Subsystem  TreatAsAtomicUnit=on
  If Action Subsystem1 : Subsystem  TreatAsAtomicUnit=on
  Merge : Merge
  Sum : Sum  Inputs=|+-
  wheel_speed : Outport
  wires:
  Sum/1 -> If Action Subsystem/1(In1), If Action Subsystem1/1(In1)
  Delay/1 -> Sum/2
  dt_change_wheel_pose/1 -> If/1, If Action Subsystem/2(dt_data_change)
  If Action Subsystem/1(Out1) -> Merge/1
  If Action Subsystem1/1(Out1) -> Merge/2
  wheel_pose_current/1 -> Sum/1, Delay/1
  If/2 -> If Action Subsystem1/Action
  If/1 -> If Action Subsystem/Action
  Merge/1 -> wheel_speed/1

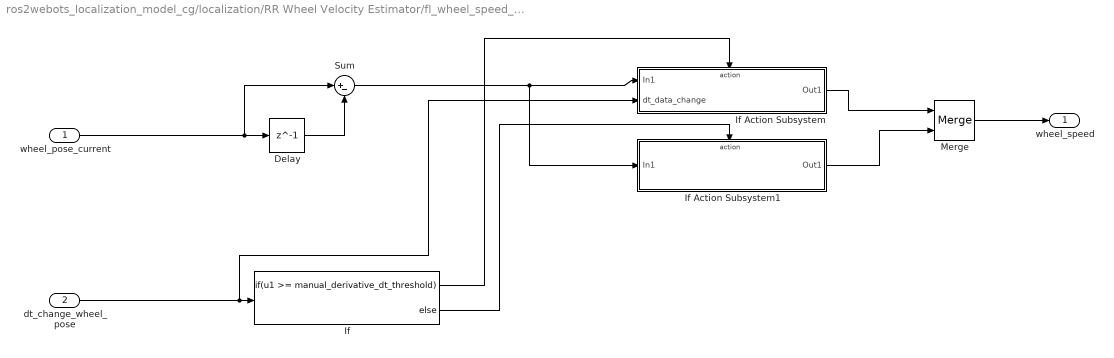
== system ros2webots_localization_model_cg/localization/RR Wheel Velocity Estimator/fl_wheel_speed_calc ==
  wheel_pose_current : Inport
  dt_change_wheel_pose : Inport  Port=2
  Delay : Delay  DelayLength=1
  If : If  IfExpression=u1 >= manual_derivative_dt_threshold
  If Action Subsystem : Subsystem  TreatAsAtomicUnit=on
  If Action Subsystem1 : Subsystem  TreatAsAtomicUnit=on
  Merge : Merge
  Sum : Sum  Inputs=|+-
  wheel_speed : Outport
  wires:
  Sum/1 -> If Action Subsystem/1(In1), If Action Subsystem1/1(In1)
  Delay/1 -> Sum/2
  dt_change_wheel_pose/1 -> If/1, If Action Subsystem/2(dt_data_change)
  If Action Subsystem/1(Out1) -> Merge/1
  If Action Subsystem1/1(Out1) -> Merge/2
  wheel_pose_current/1 -> Sum/1, Delay/1
  If/2 -> If Action Subsystem1/Action
  If/1 -> If Action Subsystem/Action
  Merge/1 -> wheel_speed/1

== system ros2webots_localization_model_cg/localization/FL Wheel Velocity Estimator/fl_wheel_speed_calc/If Action Subsystem ==
  In1 : Inport
  dt_data_change : Inport  Port=2
  Action Port : ActionPort  ActionPortLabel=if(u1 >= manual_derivative_dt_threshold)
  Divide : Product  Inputs=*/
  Out1 : Outport
  wires:
  In1/1 -> Divide/1
  dt_data_change/1 -> Divide/2
  Divide/1 -> Out1/1

== system ros2webots_localization_model_cg/localization/FL Wheel Velocity Estimator/fl_wheel_speed_calc/If Action Subsystem1 ==
  In1 : Inport
  Action Port : ActionPort  ActionPortLabel=else
  Out1 : Outport
  wires:
  In1/1 -> Out1/1

== system ros2webots_localization_model_cg/localization/FR Wheel Velocity Estimator/fl_wheel_speed_calc/If Action Subsystem ==
  In1 : Inport
  dt_data_change : Inport  Port=2
  Action Port : ActionPort  ActionPortLabel=if(u1 >= manual_derivative_dt_threshold)
  Divide : Product  Inputs=*/
  Out1 : Outport
  wires:
  In1/1 -> Divide/1
  dt_data_change/1 -> Divide/2
  Divide/1 -> Out1/1

== system ros2webots_localization_model_cg/localization/FR Wheel Velocity Estimator/fl_wheel_speed_calc/If Action Subsystem1 ==
  In1 : Inport
  Action Port : ActionPort  ActionPortLabel=else
  Out1 : Outport
  wires:
  In1/1 -> Out1/1

== system ros2webots_localization_model_cg/localization/RL Wheel Velocity Estimator/fl_wheel_speed_calc/If Action Subsystem ==
  In1 : Inport
  dt_data_change : Inport  Port=2
  Action Port : ActionPort  ActionPortLabel=if(u1 >= manual_derivative_dt_threshold)
  Divide : Product  Inputs=*/
  Out1 : Outport
  wires:
  In1/1 -> Divide/1
  dt_data_change/1 -> Divide/2
  Divide/1 -> Out1/1

== system ros2webots_localization_model_cg/localization/RL Wheel Velocity Estimator/fl_wheel_speed_calc/If Action Subsystem1 ==
  In1 : Inport
  Action Port : ActionPort  ActionPortLabel=else
  Out1 : Outport
  wires:
  In1/1 -> Out1/1

== system ros2webots_localization_model_cg/localization/RR Wheel Velocity Estimator/fl_wheel_speed_calc/If Action Subsystem ==
  In1 : Inport
  dt_data_change : Inport  Port=2
  Action Port : ActionPort  ActionPortLabel=if(u1 >= manual_derivative_dt_threshold)
  Divide : Product  Inputs=*/
  Out1 : Outport
  wires:
  In1/1 -> Divide/1
  dt_data_change/1 -> Divide/2
  Divide/1 -> Out1/1

== system ros2webots_localization_model_cg/localization/RR Wheel Velocity Estimator/fl_wheel_speed_calc/If Action Subsystem1 ==
  In1 : Inport
  Action Port : ActionPort  ActionPortLabel=else
  Out1 : Outport
  wires:
  In1/1 -> Out1/1
